simulink model "ENME562_Lab4_PID_Tanks_2022b"  (R2023a)
settings: Solver=ode1  StartTime=0.0  StopTime=30  FixedStep=0.001  RelTol=1e-3  EnableMultiTasking=on
libraries: simulink x1
settings Model: ExtModeTrigDuration=10000  Creator=smutbox  LastModifiedBy=smutbox
settings SolverCC: AlgebraicLoopSolver=TrustRegion  PositivePriorityOrder=on
settings OptimizationCC: LifeSpan=inf
settings DebuggingCC: UnconnectedInputMsg=warning  UnconnectedOutputMsg=warning  UnconnectedLineMsg=warning  ArithmeticOperatorsInVariantConditions=warning
settings ModelReferenceCC: EnableRefExpFcnMdlSchedulingChecks=on
settings SFSimCC: SimUseLocalCustomCode=off  CustomCodeUndefinedFunction=UseInterfaceOnly
settings RTWCC: Description=QUARC Win64 Target  SystemTargetFile=quarc_win64.tlc  TemplateMakefile=quarc_default_tmf  RTWUseLocalCustomCode=off  DLArmComputeVersion=19.05
settings CodeAppCC: StateflowObjectComments=on
settings STFCustomTargetCC: TargetPreCompLibLocation=C:\PROGRA~3\QUARC\lib\2016a\win64\release  UseToolchainInfoCompliant=off  SystemTargetFile=quarc_win64.tlc
settings GRTTargetCC: TargetPreCompLibLocation=C:\PROGRA~3\QUARC\lib\2016a\win64\release  ParMdlRefBuildCompliant=off  CompOptLevelCompliant=off  CombineOutputUpdateFcns=off  MatFileLogging=off  CPPClassGenCompliant=off  GRTInterface=on  UseToolchainInfoCompliant=off  ExtMode=on  ExtModeMexFile=quarc_comm
settings ConfigComp: CovMetricSettings=dswe

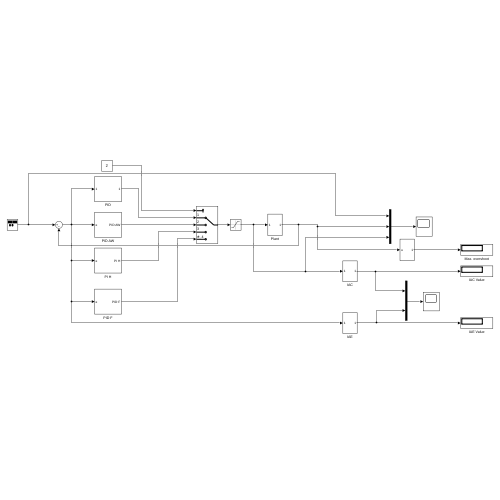
[thumbnail: Simulink's stored preview of the top-level diagram]
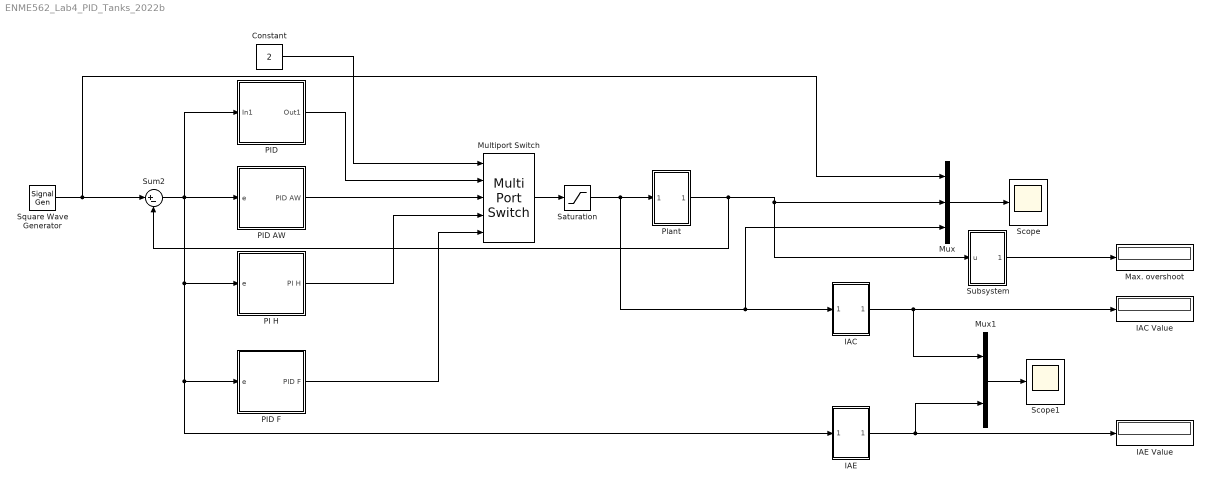
== system ENME562_Lab4_PID_Tanks_2022b ==
  Constant : Constant  Value=2
  IAC : Subsystem
  IAC Value : Display
  IAE : Subsystem
  IAE Value : Display
  Max. overshoot : Display
  Multiport Switch : MultiPortSwitch  Inputs=4  SaturateOnIntegerOverflow=off  InputSameDT=off
  Mux : Mux  Inputs=3
  Mux1 : Mux  Inputs=2
  PI H : Subsystem
  PID : Subsystem
  PID AW : Subsystem
  PID F : Subsystem
  Plant : Subsystem
  Saturation : Saturate  UpperLimit=10  LowerLimit=-10
  Scope : Scope
  Scope1 : Scope
  Square Wave Generator : SignalGenerator  WaveForm=square  Amplitude=5  Frequency=0.2  Units=rad/sec
  Subsystem : Subsystem
  Sum2 : Sum  Inputs=|+-
  wires:
  Subsystem/1(Out1) -> Max. overshoot/1
  Plant/1(Out1) -> Sum2/2, Subsystem/1(u), Mux/2
  IAC/1(Out1) -> Mux1/1, IAC Value/1
  Sum2/1 -> PID/1(In1), IAE/1(In1), PID F/1(e), PI H/1(e), PID AW/1(e)
  PID F/1(PID F) -> Multiport Switch/5
  PI H/1(PI H) -> Multiport Switch/4
  PID AW/1(PID AW) -> Multiport Switch/3
  Mux1/1 -> Scope1/1
  Constant/1 -> Multiport Switch/1
  PID/1(Out1) -> Multiport Switch/2
  Mux/1 -> Scope/1
  Multiport Switch/1 -> Saturation/1
  Saturation/1 -> Mux/3, IAC/1(In1), Plant/1(In1)
  IAE/1(Out1) -> Mux1/2, IAE Value/1
  Square Wave Generator/1 -> Mux/1, Sum2/1

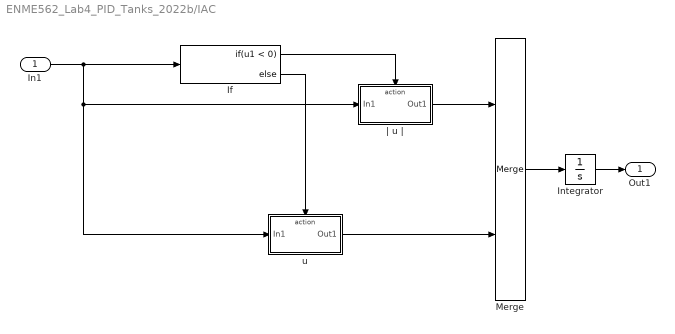
== system ENME562_Lab4_PID_Tanks_2022b/IAC ==
  In1 : Inport
  If : If  IfExpression=u1 < 0
  Integrator : Integrator
  Merge : Merge
  u : Subsystem  TreatAsAtomicUnit=on
  | u | : Subsystem  TreatAsAtomicUnit=on
  Out1 : Outport
  wires:
  If/1 -> | u |/Action
  If/2 -> u/Action
  In1/1 -> u/1(In1), | u |/1(In1), If/1
  u/1(Out1) -> Merge/2
  Merge/1 -> Integrator/1
  | u |/1(Out1) -> Merge/1
  Integrator/1 -> Out1/1

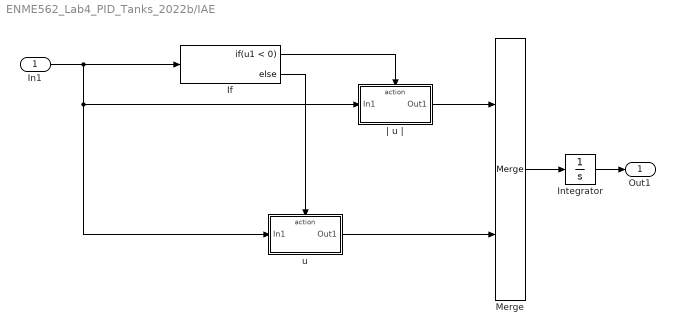
== system ENME562_Lab4_PID_Tanks_2022b/IAE ==
  In1 : Inport
  If : If  IfExpression=u1 < 0
  Integrator : Integrator
  Merge : Merge
  u : Subsystem  TreatAsAtomicUnit=on
  | u | : Subsystem  TreatAsAtomicUnit=on
  Out1 : Outport
  wires:
  If/1 -> | u |/Action
  If/2 -> u/Action
  In1/1 -> u/1(In1), | u |/1(In1), If/1
  u/1(Out1) -> Merge/2
  Merge/1 -> Integrator/1
  | u |/1(Out1) -> Merge/1
  Integrator/1 -> Out1/1

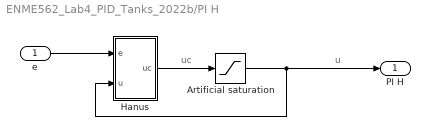
== system ENME562_Lab4_PID_Tanks_2022b/PI H ==
  note: u
  note: uc
  e : Inport
  Artificial saturation : Saturate  UpperLimit=10  LowerLimit=-10
  Hanus : Subsystem
  PI H : Outport  VectorParamsAs1DForOutWhenUnconnected=off
  wires:
  Artificial saturation/1 -> Hanus/2(u), PI H/1
  Hanus/1(uc) -> Artificial saturation/1
  e/1 -> Hanus/1(e)

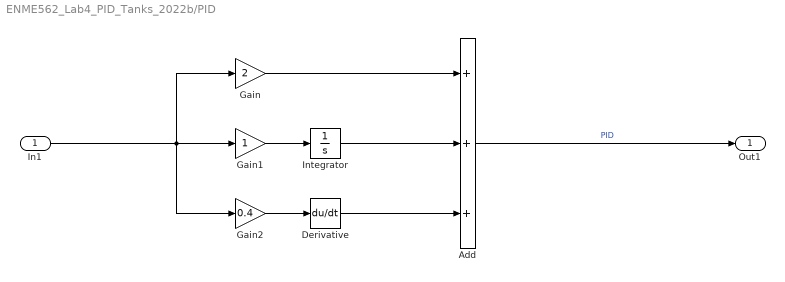
== system ENME562_Lab4_PID_Tanks_2022b/PID ==
  In1 : Inport
  Add : Sum  Inputs=+++
  Derivative : Derivative
  Gain : Gain  Gain=2
  Gain1 : Gain
  Gain2 : Gain  Gain=0.4
  Integrator : Integrator
  Out1 : Outport
  wires:
  Gain2/1 -> Derivative/1
  Gain/1 -> Add/1
  Derivative/1 -> Add/3
  Integrator/1 -> Add/2
  Gain1/1 -> Integrator/1
  Add/1 -> Out1/1  "PID"
  In1/1 -> Gain2/1, Gain1/1, Gain/1

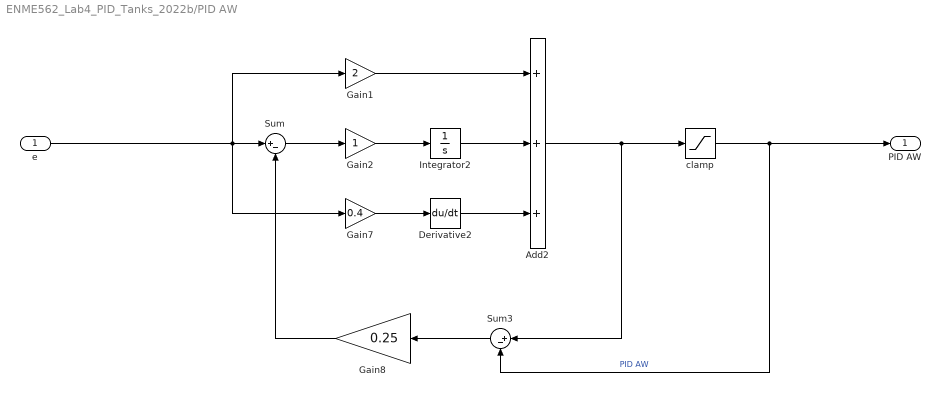
== system ENME562_Lab4_PID_Tanks_2022b/PID AW ==
  e : Inport
  Add2 : Sum  Inputs=+++
  Derivative2 : Derivative
  Gain1 : Gain  Gain=2
  Gain2 : Gain
  Gain7 : Gain  Gain=0.4
  Gain8 : Gain  Gain=0.25
  Integrator2 : Integrator
  Sum : Sum  Inputs=|+-
  Sum3 : Sum  Inputs=|+-
  clamp : Saturate  UpperLimit=10  LowerLimit=-10
  PID AW : Outport  VectorParamsAs1DForOutWhenUnconnected=off
  wires:
  e/1 -> Sum/1, Gain1/1, Gain7/1
  Sum/1 -> Gain2/1
  Integrator2/1 -> Add2/2
  Gain7/1 -> Derivative2/1
  clamp/1 -> PID AW/1, Sum3/2  "PID AW"
  Gain2/1 -> Integrator2/1
  Derivative2/1 -> Add2/3
  Gain1/1 -> Add2/1
  Add2/1 -> Sum3/1, clamp/1
  Gain8/1 -> Sum/2
  Sum3/1 -> Gain8/1

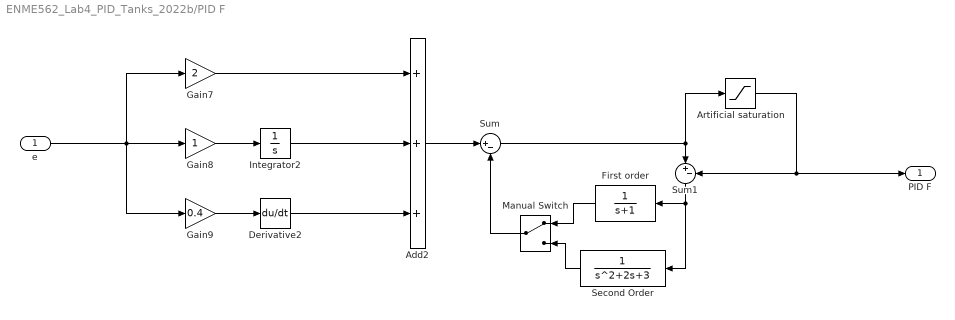
== system ENME562_Lab4_PID_Tanks_2022b/PID F ==
  e : Inport
  Add2 : Sum  Inputs=+++
  Artificial saturation : Saturate  UpperLimit=10  LowerLimit=-10
  Derivative2 : Derivative
  First order : TransferFcn  Denominator=[1 1]
  Gain7 : Gain  Gain=2
  Gain8 : Gain
  Gain9 : Gain  Gain=0.4
  Integrator2 : Integrator
  Manual Switch : ManualSwitch
  Second Order : TransferFcn  Denominator=[1 2 3]
  Sum : Sum  Inputs=|+-
  Sum1 : Sum  Inputs=|+-
  PID F : Outport  VectorParamsAs1DForOutWhenUnconnected=off
  wires:
  e/1 -> Gain9/1, Gain8/1, Gain7/1
  Gain7/1 -> Add2/1
  Integrator2/1 -> Add2/2
  Gain8/1 -> Integrator2/1
  Derivative2/1 -> Add2/3
  Gain9/1 -> Derivative2/1
  Artificial saturation/1 -> PID F/1, Sum1/2
  Add2/1 -> Sum/1
  Sum/1 -> Sum1/1, Artificial saturation/1
  Sum1/1 -> First order/1, Second Order/1
  First order/1 -> Manual Switch/1
  Second Order/1 -> Manual Switch/2
  Manual Switch/1 -> Sum/2

== system ENME562_Lab4_PID_Tanks_2022b/Plant ==
  In1 : Inport
  Out1 : Outport

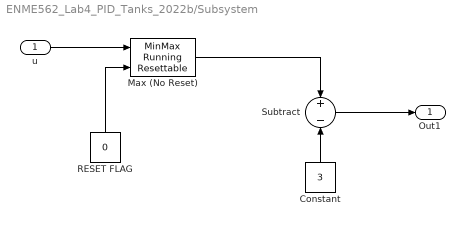
== system ENME562_Lab4_PID_Tanks_2022b/Subsystem ==
  u : Inport
  Constant : Constant  Value=3
  Max (No Reset) : simulink/Math Operations/MinMax Running Resettable  Function=max  vinit=0.0
  RESET FLAG : Constant  Value=0
  Subtract : Sum  Inputs=+-
  Out1 : Outport
  wires:
  Constant/1 -> Subtract/2
  Max (No Reset)/1 -> Subtract/1
  Subtract/1 -> Out1/1
  u/1 -> Max (No Reset)/1
  RESET FLAG/1 -> Max (No Reset)/2

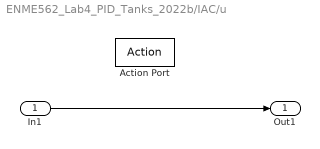
== system ENME562_Lab4_PID_Tanks_2022b/IAC/u ==
  In1 : Inport
  Action Port : ActionPort  ActionPortLabel=else
  Out1 : Outport
  wires:
  In1/1 -> Out1/1

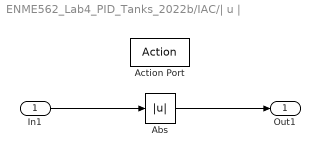
== system ENME562_Lab4_PID_Tanks_2022b/IAC/| u | ==
  In1 : Inport
  Action Port : ActionPort  ActionPortLabel=if(u1 < 0)
  Abs : Abs  SaturateOnIntegerOverflow=off
  Out1 : Outport
  wires:
  In1/1 -> Abs/1
  Abs/1 -> Out1/1

== system ENME562_Lab4_PID_Tanks_2022b/IAE/u ==
  In1 : Inport
  Action Port : ActionPort  ActionPortLabel=else
  Out1 : Outport
  wires:
  In1/1 -> Out1/1

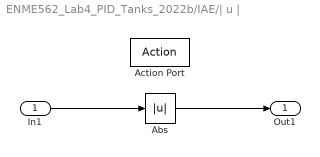
== system ENME562_Lab4_PID_Tanks_2022b/IAE/| u | ==
  In1 : Inport
  Action Port : ActionPort  ActionPortLabel=if(u1 < 0)
  Abs : Abs  SaturateOnIntegerOverflow=off
  Out1 : Outport
  wires:
  In1/1 -> Abs/1
  Abs/1 -> Out1/1

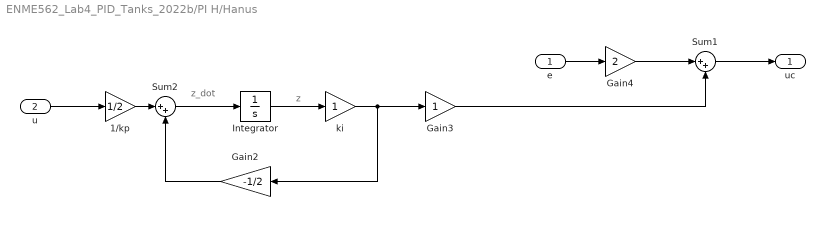
== system ENME562_Lab4_PID_Tanks_2022b/PI H/Hanus ==
  note: z_dot
  note: z
  e : Inport
  u : Inport  Port=2
  1/kp : Gain  Gain=1/2
  Gain2 : Gain  Gain=-1/2
  Gain3 : Gain
  Gain4 : Gain  Gain=2
  Integrator : Integrator
  Sum1 : Sum  Inputs=|++
  Sum2 : Sum  Inputs=|++
  ki : Gain
  uc : Outport
  wires:
  Gain3/1 -> Sum1/2
  e/1 -> Gain4/1
  ki/1 -> Gain2/1, Gain3/1
  Gain4/1 -> Sum1/1
  Integrator/1 -> ki/1
  Sum1/1 -> uc/1
  u/1 -> 1/kp/1
  1/kp/1 -> Sum2/1
  Sum2/1 -> Integrator/1
  Gain2/1 -> Sum2/2
